simulink model "heli_quanser_base"  (R2025a)
settings: Solver=FixedStepAuto  StartTime=0.0  StopTime=30  FixedStep=0.001  RelTol=1e-3  EnableMultiTasking=on
values from neighbouring files (symbols this model uses):
  theta_0 = -40.5*pi/180    (= -0.706858347058)    [setup_heli_2d_base.m]
  Ts = Gz_inestable.Ts    [minimosCuadrados.m]    (also in minimosCuadradosMIMO.m = Gz_in.Ts; setup_heli_2d_base.m = 0.001)
  VMAX_UPM_P = 24    [setup_heli_2d_base.m]
  VMAX_UPM_Y = 15    [setup_heli_2d_base.m]
undefined symbols (not defined in the file or in its folder): B_p, B_y, g, J_eq_p, J_eq_y, K_pp, K_py, K_yp, K_yy, l_cm, m_heli
libraries: simulink x2, simulink_extras x1
settings Model: Creator=Jorge Romero  LastModifiedBy=ingem
settings SolverCC: AlgebraicLoopSolver=TrustRegion
settings DataIOCC: LimitDataPoints=on  SaveFormat=Array  ReturnWorkspaceOutputs=off
settings OptimizationCC: ExpressionDepthLimit=2147483647.0  LifeSpan=inf
settings DebuggingCC: UnderspecifiedInitializationDetection=Classic  MergeDetectMultiDrivingBlocksExec=none  SolverPrmCheckMsg=warning  UnconnectedInputMsg=warning  UnconnectedOutputMsg=warning  UnconnectedLineMsg=warning  StateNameClashWarn=warning  SFUnexpectedBacktrackingDiag=warning  SFNoUnconditionalDefaultTransitionDiag=warning  SFExecutionAtInitializationDiag=none  ArithmeticOperatorsInVariantConditions=warning
settings HardwareCC: ProdBitPerPointer=32.0  ProdBitPerSizeT=32.0  ProdBitPerPtrDiffT=32.0  ProdLargestAtomicFloat=None  ProdIntDivRoundTo=Undefined  ProdEndianess=Unspecified  ProdWordSize=32.0  ProdHWDeviceType=32-bit Generic
settings ModelReferenceCC: EnableRefExpFcnMdlSchedulingChecks=on  PropagateSignalLabelsOutOfModel=off
settings SFSimCC: SimUseLocalCustomCode=off  CustomCodeUndefinedFunction=UseInterfaceOnly
settings RTWCC: RTWUseLocalCustomCode=off  GPUComputeCapability=3.5  DLArmComputeVersion=19.05
settings CodeAppCC: StateflowObjectComments=on
settings GRTTargetCC: TargetLangStandard=C89/C90 (ANSI)
settings ConfigComp: CovMetricSettings=dw  CovSaveCumulativeToWorkspaceVar=on  CovSaveSingleToWorkspaceVar=on  CovExternalEMLEnable=off

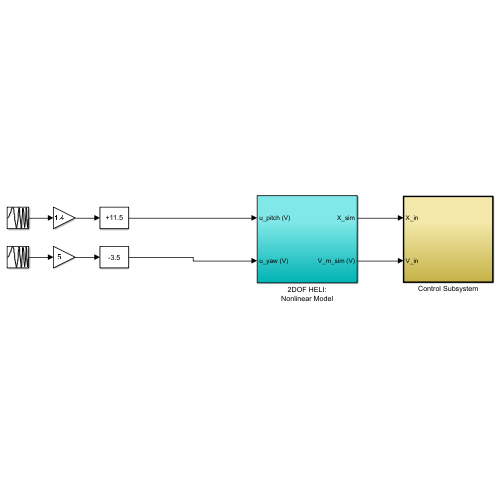
[thumbnail: Simulink's stored preview of the top-level diagram]
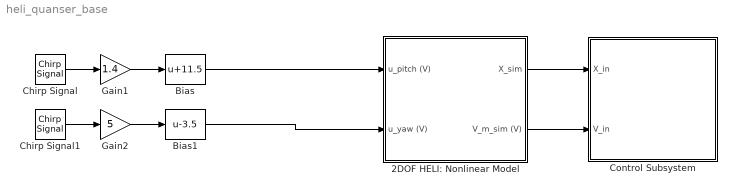
== system heli_quanser_base ==
  2DOF HELI: Nonlinear Model : Subsystem
  Bias : Bias  Bias=11.5  SaturateOnIntegerOverflow=off
  Bias1 : Bias  Bias=-3.5  SaturateOnIntegerOverflow=off
  Chirp Signal : simulink/Sources/Chirp Signal  f1=0.08  T=10  f2=1
  Chirp Signal1 : simulink/Sources/Chirp Signal  f1=0.05  T=100  f2=1
  Control Subsystem : Subsystem  TreatAsAtomicUnit=on
  Gain1 : Gain  Gain=1.4
  Gain2 : Gain  Gain=5
  wires:
  Gain2/1 -> Bias1/1
  Gain1/1 -> Bias/1
  Chirp Signal1/1 -> Gain2/1
  Chirp Signal/1 -> Gain1/1
  Bias/1 -> 2DOF HELI: Nonlinear Model/1(u_pitch (V))
  Bias1/1 -> 2DOF HELI: Nonlinear Model/2(u_yaw (V))
  2DOF HELI: Nonlinear Model/1(X_sim) -> Control Subsystem/1(X_in)
  2DOF HELI: Nonlinear Model/2(V_m_sim (V)) -> Control Subsystem/2(V_in)

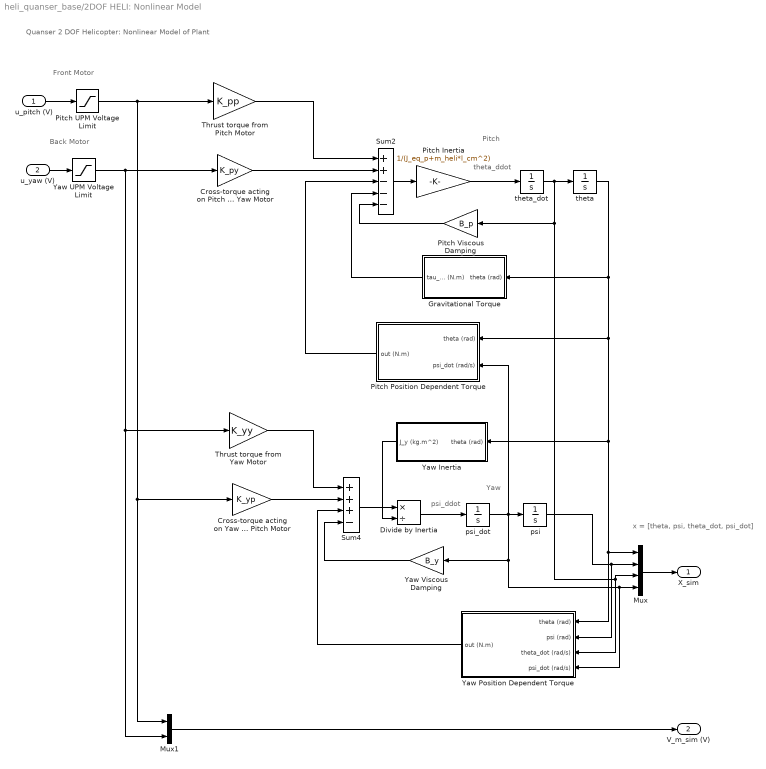
== system heli_quanser_base/2DOF HELI: Nonlinear Model ==
  note: Back Motor
  note: Front Motor
  note: x = [theta, psi, theta_dot, psi_dot]
  note: Quanser 2 DOF Helicopter: Nonlinear Model of Plant
  note: theta_ddot
  note: psi_ddot
  note: Pitch
  note: Yaw
  u_pitch (V) : Inport
  u_yaw (V) : Inport  Port=2
  Cross-torque acting on Pitch from Yaw Motor : Gain  Gain=K_py
  Cross-torque acting on Yaw from Pitch Motor : Gain  Gain=K_yp
  Divide by Inertia : Product  Inputs=*/
  Gravitational Torque : Subsystem
  Mux : Mux
  Mux1 : Mux  Inputs=2
  Pitch Inertia : Gain  Gain=1/(J_eq_p+m_heli*l_cm^2)
  Pitch Position Dependent Torque : Subsystem  AncestorBlock=heli_2d_lib/2DOF Helicopter: Nonlinear Model/Yaw Nonlinear Element
  Pitch UPM Voltage Limit : Saturate  UpperLimit=VMAX_UPM_P  LowerLimit=- VMAX_UPM_P
  Pitch Viscous Damping : Gain  Gain=B_p
  Sum2 : Sum  Inputs=++---
  Sum4 : Sum  Inputs=+++-
  Thrust torque from Pitch Motor : Gain  Gain=K_pp
  Thrust torque from Yaw Motor : Gain  Gain=K_yy
  Yaw Inertia : Subsystem
  Yaw Position Dependent Torque : Subsystem
  Yaw UPM Voltage Limit : Saturate  UpperLimit=VMAX_UPM_Y  LowerLimit=- VMAX_UPM_Y
  Yaw Viscous Damping : Gain  Gain=B_y
  psi : Integrator
  psi_dot : Integrator
  theta : Integrator  InitialCondition=theta_0  LimitOutput=on  UpperSaturationLimit=40.5*pi/180  LowerSaturationLimit=-40.5*pi/180
  theta_dot : Integrator
  X_sim : Outport
  V_m_sim (V) : Outport  Port=2
  wires:
  Pitch Position Dependent Torque/1(out (N.m)) -> Sum2/3
  Gravitational Torque/1(tau_g (N.m)) -> Sum2/4
  Pitch Viscous Damping/1 -> Sum2/5
  Cross-torque acting on Pitch from Yaw Motor/1 -> Sum2/2
  Thrust torque from Pitch Motor/1 -> Sum2/1
  Yaw Inertia/1(J_y (kg.m^2)) -> Divide by Inertia/2
  Divide by Inertia/1 -> psi_dot/1
  Sum4/1 -> Divide by Inertia/1
  Yaw Position Dependent Torque/1(out (N.m)) -> Sum4/3
  Yaw Viscous Damping/1 -> Sum4/4
  psi/1 -> Yaw Position Dependent Torque/2(psi (rad)), Mux/2
  Mux1/1 -> V_m_sim (V)/1
  Yaw UPM Voltage Limit/1 -> Thrust torque from Yaw Motor/1, Mux1/2, Cross-torque acting on Pitch from Yaw Motor/1
  Pitch UPM Voltage Limit/1 -> Mux1/1, Cross-torque acting on Yaw from Pitch Motor/1, Thrust torque from Pitch Motor/1
  Mux/1 -> X_sim/1
  theta/1 -> Gravitational Torque/1(theta (rad)), Pitch Position Dependent Torque/1(theta (rad)), Yaw Position Dependent Torque/1(theta (rad)), Mux/1, Yaw Inertia/1(theta (rad))
  Sum2/1 -> Pitch Inertia/1
  Pitch Inertia/1 -> theta_dot/1
  theta_dot/1 -> Pitch Viscous Damping/1, Yaw Position Dependent Torque/3(theta_dot (rad/s)), Mux/3, theta/1
  Thrust torque from Yaw Motor/1 -> Sum4/1
  Cross-torque acting on Yaw from Pitch Motor/1 -> Sum4/2
  psi_dot/1 -> Yaw Viscous Damping/1, Yaw Position Dependent Torque/4(psi_dot (rad/s)), Mux/4, Pitch Position Dependent Torque/2(psi_dot (rad/s)), psi/1
  u_pitch (V)/1 -> Pitch UPM Voltage Limit/1
  u_yaw (V)/1 -> Yaw UPM Voltage Limit/1

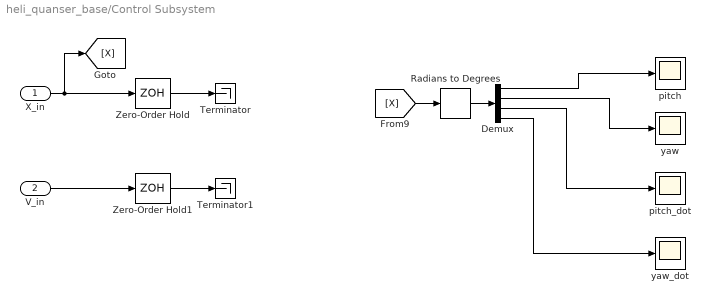
== system heli_quanser_base/Control Subsystem ==
  X_in : Inport
  V_in : Inport  Port=2
  Demux : Demux
      settings: DisplayOption=none
  Radians to Degrees : simulink_extras/Transformations/Radians to Degrees
  Terminator : Terminator
  Terminator1 : Terminator
  Zero-Order Hold : ZeroOrderHold  SampleTime=Ts
  Zero-Order Hold1 : ZeroOrderHold  SampleTime=Ts
  pitch : Scope
      settings: TimeSpan=30  ActiveDisplayYMinimum=-81.99762  ActiveDisplayYMaximum=9.11085
  pitch_dot : Scope
      settings: TimeSpan=30  ActiveDisplayYMinimum=-48.65452  ActiveDisplayYMaximum=62.46494
  yaw : Scope
      settings: TimeSpan=30  ActiveDisplayYMinimum=-31.83031  ActiveDisplayYMaximum=286.47281  DataLoggingVariableName=ScopeData2
  yaw_dot : Scope
      settings: TimeSpan=30  ActiveDisplayYMinimum=-83.27416  ActiveDisplayYMaximum=83.72639  DataLoggingVariableName=ScopeData3
  wires:
  X_in/1 -> [X], Zero-Order Hold/1
  V_in/1 -> Zero-Order Hold1/1
  Demux/1 -> pitch/1
  Demux/4 -> yaw_dot/1
  Radians to Degrees/1 -> Demux/1
  [X] -> Radians to Degrees/1
  Demux/3 -> pitch_dot/1
  Demux/2 -> yaw/1
  Zero-Order Hold/1 -> Terminator/1
  Zero-Order Hold1/1 -> Terminator1/1

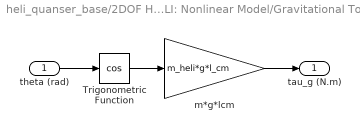
== system heli_quanser_base/2DOF HELI: Nonlinear Model/Gravitational Torque ==
  theta (rad) : Inport
  Trigonometric Function : Trigonometry  Operator=cos  OutputSignalType=real
  m*g*lcm : Gain  Gain=m_heli*g*l_cm
  tau_g (N.m) : Outport
  wires:
  m*g*lcm/1 -> tau_g (N.m)/1
  theta (rad)/1 -> Trigonometric Function/1
  Trigonometric Function/1 -> m*g*lcm/1

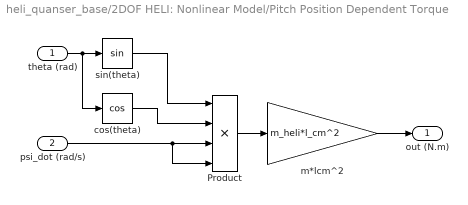
== system heli_quanser_base/2DOF HELI: Nonlinear Model/Pitch Position Dependent Torque ==
  theta (rad) : Inport
  psi_dot (rad/s) : Inport  Port=2
  Product : Product  Inputs=4  RndMeth=Zero
  cos(theta) : Trigonometry  Operator=cos  OutputSignalType=real
  m*lcm^2 : Gain  Gain=m_heli*l_cm^2
  sin(theta) : Trigonometry  OutputSignalType=real
  out (N.m) : Outport
  wires:
  psi_dot (rad/s)/1 -> Product/4, Product/3
  theta (rad)/1 -> cos(theta)/1, sin(theta)/1
  Product/1 -> m*lcm^2/1
  sin(theta)/1 -> Product/1
  cos(theta)/1 -> Product/2
  m*lcm^2/1 -> out (N.m)/1

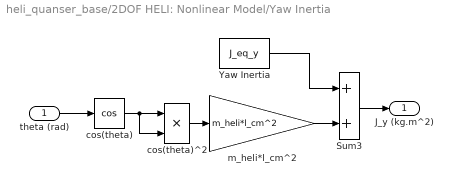
== system heli_quanser_base/2DOF HELI: Nonlinear Model/Yaw Inertia ==
  theta (rad) : Inport
  Sum3 : Sum
  Yaw Inertia : Constant  Value=J_eq_y
  cos(theta) : Trigonometry  Operator=cos  OutputSignalType=real
  cos(theta)^2 : Product  RndMeth=Zero
  m_heli*l_cm^2 : Gain  Gain=m_heli*l_cm^2
  J_y (kg.m^2) : Outport
  wires:
  cos(theta)/1 -> cos(theta)^2/2, cos(theta)^2/1
  Sum3/1 -> J_y (kg.m^2)/1
  theta (rad)/1 -> cos(theta)/1
  m_heli*l_cm^2/1 -> Sum3/2
  Yaw Inertia/1 -> Sum3/1
  cos(theta)^2/1 -> m_heli*l_cm^2/1

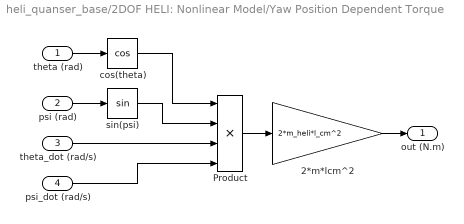
== system heli_quanser_base/2DOF HELI: Nonlinear Model/Yaw Position Dependent Torque ==
  theta (rad) : Inport
  psi (rad) : Inport  Port=2
  theta_dot (rad/s) : Inport  Port=3
  psi_dot (rad/s) : Inport  Port=4
  2*m*lcm^2 : Gain  Gain=2*m_heli*l_cm^2
  Product : Product  Inputs=4  RndMeth=Zero
  cos(theta) : Trigonometry  Operator=cos  OutputSignalType=real
  sin(psi) : Trigonometry  OutputSignalType=real
  out (N.m) : Outport
  wires:
  2*m*lcm^2/1 -> out (N.m)/1
  psi_dot (rad/s)/1 -> Product/4
  theta_dot (rad/s)/1 -> Product/3
  sin(psi)/1 -> Product/2
  cos(theta)/1 -> Product/1
  Product/1 -> 2*m*lcm^2/1
  theta (rad)/1 -> cos(theta)/1
  psi (rad)/1 -> sin(psi)/1
